simulink model "FuelCell"  (R2023a)
settings: Solver=VariableStepAuto  StartTime=0.0  StopTime=10  RelTol=1e-3
libraries: simulink x1, spspowerguiLib x1
settings Model: Creator=pc  LastModifiedBy=Faraz
settings DebuggingCC: ParameterPrecisionLossMsg=none

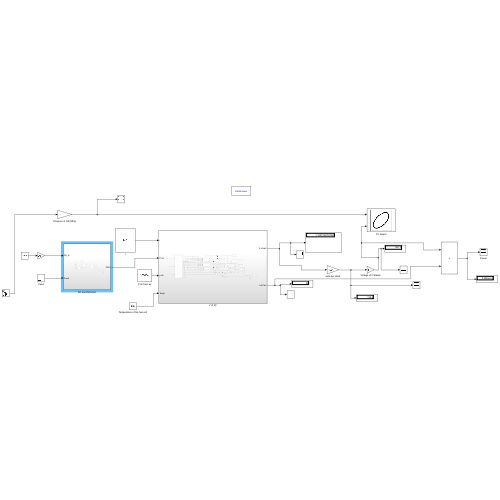
[thumbnail: Simulink's stored preview of the top-level diagram]
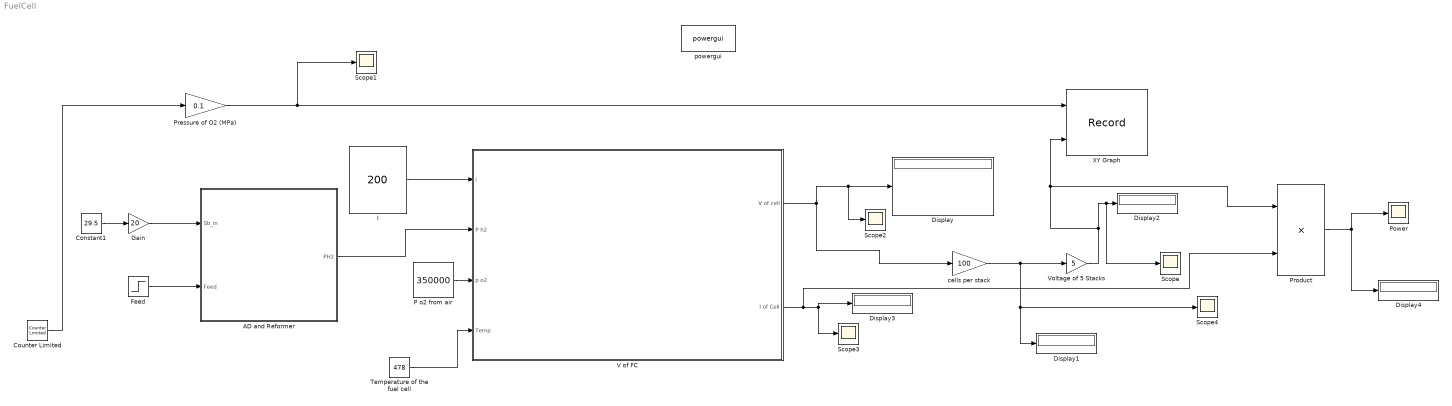
== system FuelCell ==
  AD and Reformer : Subsystem
  Constant1 : Constant  Value=29.5
  Counter Limited : simulink/Sources/Counter Limited  uplimit=50  tsamp=-1
  Display{,1..4} (5 alike) : Display
  Feed : Step  SampleTime=0
  Gain : Gain  Gain=20
  I : Constant  Value=200
  P o2 from air : Constant  Value=350000
  Power : Scope
  Pressure of O2 (MPa) : Gain  Gain=0.1
  Product : Product
  Scope{,1..4} (5 alike) : Scope
  Temperature of the fuel cell : Constant  Value=478
  V of FC : Subsystem
  Voltage of 5 Stacks : Gain  Gain=5
  XY Graph : Record  FileSettingsInternal="{\"entries\":[{\"content\":{\"excelSettings\":{\"content\":{},\"type\":\"Streamout.ExcelSettings\"}},\"type\":\"Streamout.FileSettingStorage\",\"uuid\":\"06980113-96f1-4b0c-a215-c6c45438d7ac\"}],\"packageUris\":[\"http://schema.mathworks.com/mf0/streamout_blocks/R2020a\"],\"version\":\"1.0\"}"  Layout=[1 1]  SignalsInternal="{\"entries\":[{\"content\":{\"signals\":[{\"content\":{\"blockPath\":[\"FuelCell/XY Graph\"],\"dimensions\":[1],\"domain\":\"FuelCell/XY Graph\",\"lineColor\":\"#a2142f\",\"plots\":[1],\"port\":1,\"sid\":[\"\"],\"signalID\":456,\"signalName\":\"Pressure of O2 (MPa)\"},\"type\":\"RecordBlkView.Signal\",\"uuid\":\"e1d00316-961b-4916-b371-07965f440cbd\"},{\"content\":{\"blockPath\":[\"FuelCell/XY Graph\"],\"dimensions\":[1],\"domain\":\"FuelCell/XY Graph\",\"lineColor\":\"#139fff\",\"plots\":[1],\"port\":2,\"sid\":[\"\"],\"signalID\":460,\"signalName\":\"Voltage of 5 Stacks\"},\"type\":\"RecordBlkView.Signal\",\"uuid\":\"8fd97479-0bd7-4bc4-89e8-e46443fea8dd\"}]},\"type\":\"RecordBlkView.InputSignals\",\"uuid\":\"3637481a-cae3-4c48-904e-6dbd072400be\"}],\"packageUris\":[\"http://schema.mathworks.com/mf0/streamout_blocks/R2020a\"],\"version\":\"1.0\"}"  VisualizationBindings="{\"xyplotplugin\":{\"info\":[{\"series\":[{\"bindingParametersList\":[{\"parameter\":\"X-Axis\",\"signalID\":456,\"signalName\":\"Pressure of O2 (MPa)\"},{\"parameter\":\"Y-Axis\",\"signalID\":460,\"signalName\":\"Voltage of 5 Stacks\"}],\"seriesID\":32857}],\"subplotID\":1}]}}"  CompatibilityTag=XY
  cells per stack : Gain  Gain=100
  powergui : spspowerguiLib/powergui  Priority=1  SimulationMode=Continuous  SampleTime=50e-6  frequency=60  Iterations=50  frequencyindice=0  Pbase=100e6  ErrMax=1e-4  UnitsV=kV  UnitsW=MW  buscounter=0  FunctionMessages=off  echomessages=off  EnableUseOfTLC=off  CurrentSourceSwitches=off  DisableSnubberDevices=off  DisableRonSwitches=off  DisableVfSwitches=off  DisplayEquations=off  AutomaticDiscreteSolvers=off  SolverType=Tustin/Backward Euler (TBE)  Interpol=off  ExternalGateDelay=off  methode=off  Ts=100  x0status=blocks  SPID=on  SwTol=0  HookPort=off  NonlinearTolerance=1e-4  nMaxIteration=100  ContinueOnMaxIteration=off  RestoreLinks=warning  ResistiveCurrentMeasurement=off  Frange=[0:2:500]  Ylog=off  Xlog=on  ShowGrid=off  save=off  variable=ZData  structure=0  ZoomFFT=off  StartTime=0.0  cycles=1  DisplayStyle=1  fundamental=60  FreqAxis=off  MaxFrequency=1000  frequencyindicesteady=1  RmsSteady=1  display=off
  wires:
  V of FC/1(V of cell) -> cells per stack/1, Scope2/1, Display/1
  I/1 -> V of FC/1("i ")
  cells per stack/1 -> Scope4/1, Display1/1, Voltage of 5 Stacks/1
  Voltage of 5 Stacks/1 -> Product/1, XY Graph/2, Scope/1, Display2/1
  Temperature of the fuel cell/1 -> V of FC/4(Temp)
  Counter Limited/1 -> Pressure of O2 (MPa)/1
  Pressure of O2 (MPa)/1 -> Scope1/1, XY Graph/1
  V of FC/2(I of Cell) -> Product/2, Display3/1, Scope3/1
  Gain/1 -> AD and Reformer/1(Sb_in)
  Constant1/1 -> Gain/1
  Feed/1 -> AD and Reformer/2(Feed)
  Product/1 -> Display4/1, Power/1
  AD and Reformer/1(PH2) -> V of FC/2(P h2)
  P o2 from air/1 -> V of FC/3(p o2)

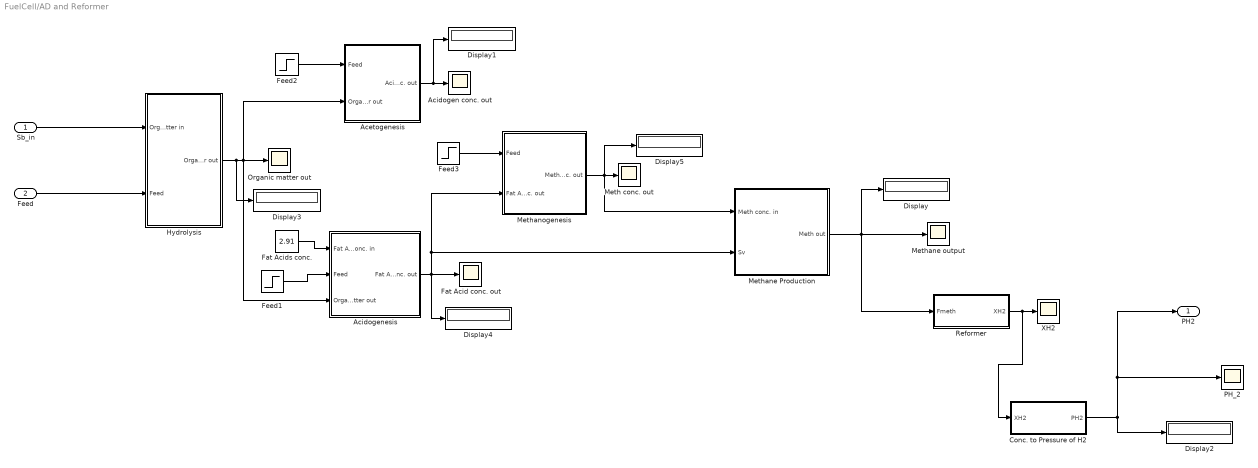
== system FuelCell/AD and Reformer ==
  Sb_in : Inport
  Feed : Inport  Port=2
  Acetogenesis : Subsystem
  Acidogen conc. out : Scope
  Acidogenesis : Subsystem
  Conc. to Pressure of H2 : Subsystem
  Display{,1..5} (6 alike) : Display
  Fat Acid conc. out : Scope
  Fat Acids conc. : Constant  Value=2.91
  Feed1 : Step  SampleTime=0
  Feed2 : Step  SampleTime=0
  Feed3 : Step  SampleTime=0
  "Hydrolysis " : Subsystem
  Meth conc. out : Scope
  Methane Production : Subsystem
  Methane output : Scope
  Methanogenesis : Subsystem
  Organic matter out : Scope
  PH_2 : Scope
  Reformer : Subsystem
  XH2 : Scope
  PH2 : Outport
  wires:
  Reformer/1(XH2) -> XH2/1, Conc. to Pressure of H2/1(XH2)
  Feed3/1 -> Methanogenesis/1(Feed)
  Feed1/1 -> Acidogenesis/2(Feed)
  Feed2/1 -> Acetogenesis/1(Feed)
  Acetogenesis/1(Acidogen conc. out) -> Display1/1, Acidogen conc. out/1
  Methanogenesis/1(Meth conc. out) -> Display5/1, Meth conc. out/1, Methane Production/1(Meth conc. in)
  Conc. to Pressure of H2/1(PH2) -> PH2/1, PH_2/1, Display2/1
  "Hydrolysis "/1(Organic matter out) -> Organic matter out/1, Acidogenesis/3(Organic matter out), Acetogenesis/2(Organic matter out), Display3/1
  Acidogenesis/1(Fat Acid conc. out) -> Display4/1, Methanogenesis/2(Fat Acid conc. out), Methane Production/2(Sv), Fat Acid conc. out/1
  Fat Acids conc./1 -> Acidogenesis/1(Fat Acid conc. in)
  Feed/1 -> "Hydrolysis "/2(Feed)
  Sb_in/1 -> "Hydrolysis "/1(Organic Matter in)
  Methane Production/1(Meth out) -> Methane output/1, Reformer/1(Fmeth), Display/1

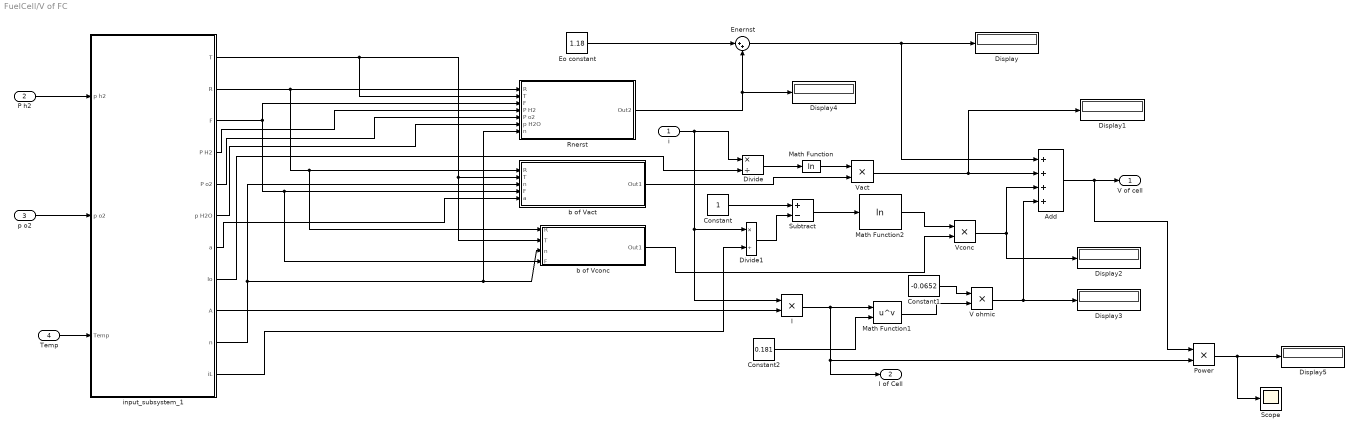
== system FuelCell/V of FC ==
  "i " : Inport
  P h2 : Inport  Port=2
  p o2 : Inport  Port=3
  Temp : Inport  Port=4
  Add : Sum  Inputs=++++
  Constant : Constant
  Constant1 : Constant  Value=-0.0652
  Constant2 : Constant  Value=0.181
  Display{,1..5} (6 alike) : Display
  Divide : Product  Inputs=*/
  Divide1 : Product  Inputs=*/
  Enernst : Sum  Inputs=|++
  "Eo constant " : Constant  Value=1.18
  I : Product
  Math Function : Math  Operator=log
  Math Function1 : Math  Operator=pow
  Math Function2 : Math  Operator=log
  Power : Product
  Rnerst : Subsystem
  Scope : Scope
  Subtract : Sum  Inputs=+-
  V ohmic : Product
  Vact : Product
  Vconc : Product
  b of Vact : Subsystem
  b of Vconc : Subsystem
  input_subsystem_1 : Subsystem
  V of cell : Outport
  I of Cell : Outport  Port=2
  wires:
  V ohmic/1 -> Display3/1, Add/4
  p o2/1 -> input_subsystem_1/2(p o2)
  input_subsystem_1/8(Io) -> Divide/2
  Temp/1 -> input_subsystem_1/3(Temp)
  P h2/1 -> input_subsystem_1/1(p h2)
  input_subsystem_1/11(iL) -> Divide1/2
  I/1 -> Math Function1/1, I of Cell/1, Power/2
  Enernst/1 -> Display/1, Add/1
  input_subsystem_1/9(A) -> I/2
  Vconc/1 -> Add/3, Display2/1
  input_subsystem_1/7(a) -> b of Vact/5(a)
  Math Function2/1 -> Vconc/1
  Constant2/1 -> Math Function1/2
  "i "/1 -> Divide/1, Divide1/1, I/1
  "Eo constant "/1 -> Enernst/1
  input_subsystem_1/5(P o2) -> Rnerst/5(P o2)
  b of Vconc/1(Out1) -> Vconc/2
  Subtract/1 -> Math Function2/1
  input_subsystem_1/6(p H2O) -> Rnerst/6(p H2O)
  input_subsystem_1/4(P H2) -> Rnerst/4(P H2)
  Constant/1 -> Subtract/1
  b of Vact/1(Out1) -> Vact/2
  Rnerst/1(Out2) -> Enernst/2, Display4/1
  Vact/1 -> Add/2, Display1/1
  Math Function/1 -> Vact/1
  Divide/1 -> Math Function/1
  input_subsystem_1/1(T) -> b of Vconc/2(T), b of Vact/2(T), Rnerst/2(T)
  Math Function1/1 -> V ohmic/2
  input_subsystem_1/2(R) -> Rnerst/1(R), b of Vconc/1(R), b of Vact/1(R)
  Add/1 -> V of cell/1, Power/1
  Divide1/1 -> Subtract/2
  Constant1/1 -> V ohmic/1
  Power/1 -> Scope/1, Display5/1
  input_subsystem_1/3(F) -> b of Vconc/4(F), b of Vact/4(F), Rnerst/3(F)
  input_subsystem_1/10(n) -> b of Vact/3(n), b of Vconc/3(n), Rnerst/7(n)

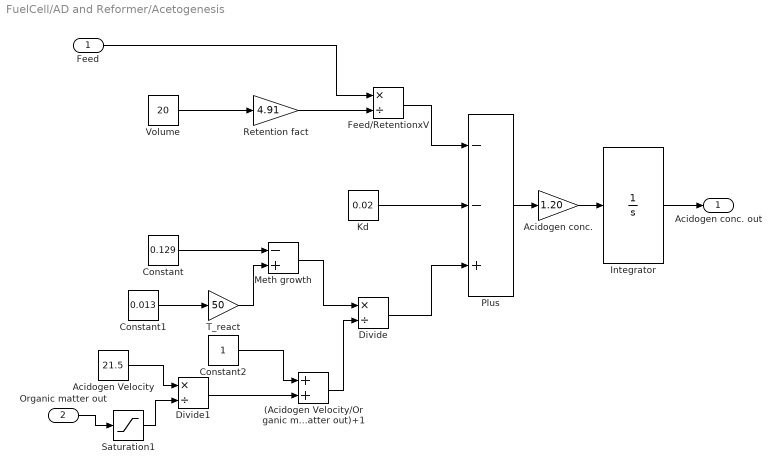
== system FuelCell/AD and Reformer/Acetogenesis ==
  Feed : Inport
  Organic matter out : Inport  Port=2
  (Acidogen Velocity/Organic matter out)+1 : Sum
  Acidogen Velocity : Constant  Value=21.5
  Acidogen conc. : Gain  Gain=1.20
  Constant : Constant  Value=0.129
  Constant1 : Constant  Value=0.013
  Constant2 : Constant
  Divide : Product  Inputs=*/
  Divide1 : Product  Inputs=*/
  Feed/RetentionxV : Product  Inputs=*/
  Integrator : Integrator
  Kd : Constant  Value=0.02
  Meth growth : Sum  Inputs=-+
  Plus : Sum  Inputs=--+
  Retention fact : Gain  Gain=4.91
  Saturation1 : Saturate  UpperLimit=300  LowerLimit=0.3
  T_react : Gain  Gain=50
  Volume : Constant  Value=20
  Acidogen conc. out : Outport
  wires:
  Volume/1 -> Retention fact/1
  Retention fact/1 -> Feed/RetentionxV/2
  Feed/1 -> Feed/RetentionxV/1
  Feed/RetentionxV/1 -> Plus/1
  Kd/1 -> Plus/2
  Acidogen conc./1 -> Integrator/1
  Plus/1 -> Acidogen conc./1
  Constant1/1 -> T_react/1
  T_react/1 -> Meth growth/2
  Constant/1 -> Meth growth/1
  Meth growth/1 -> Divide/1
  (Acidogen Velocity/Organic matter out)+1/1 -> Divide/2
  Constant2/1 -> (Acidogen Velocity/Organic matter out)+1/1
  Acidogen Velocity/1 -> Divide1/1
  Divide/1 -> Plus/3
  Integrator/1 -> Acidogen conc. out/1
  Organic matter out/1 -> Saturation1/1
  Divide1/1 -> (Acidogen Velocity/Organic matter out)+1/2
  Saturation1/1 -> Divide1/2

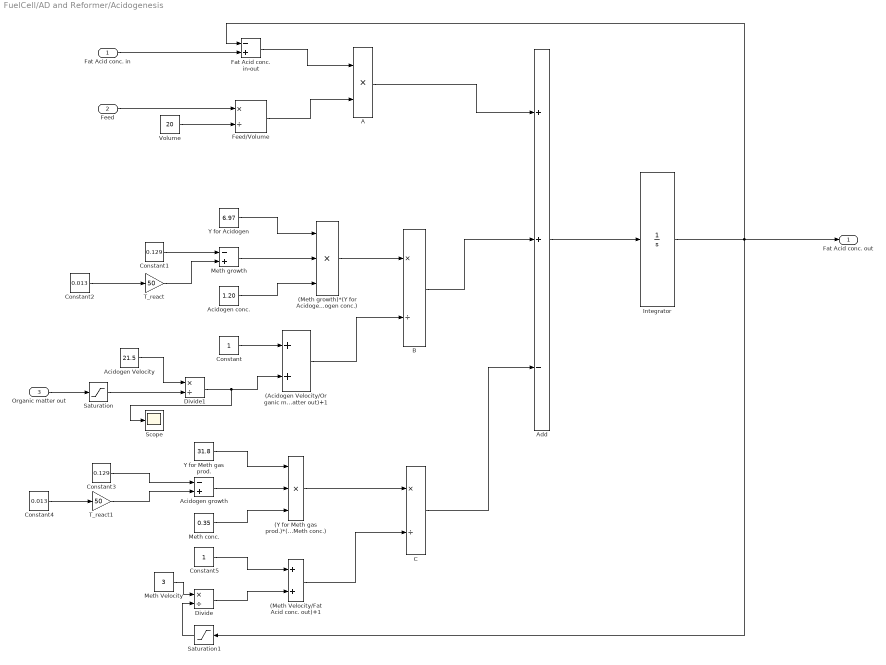
== system FuelCell/AD and Reformer/Acidogenesis ==
  Fat Acid conc. in : Inport
  Feed : Inport  Port=2
  Organic matter out : Inport  Port=3
  (Acidogen Velocity/Organic matter out)+1 : Sum
  (Meth Velocity/Fat Acid conc. out)+1 : Sum
  (Meth growth)*(Y for Acidogen)*(Acidogen conc.) : Product  Inputs=3
  (Y for Meth gas prod.)*(Acid growth)*(Meth conc.) : Product  Inputs=3
  A : Product
  Acidogen Velocity : Constant  Value=21.5
  Acidogen conc. : Constant  Value=1.20
  Acidogen growth : Sum  Inputs=-+
  Add : Sum  Inputs=++-
  B : Product  Inputs=*/
  C : Product  Inputs=*/
  Constant : Constant
  Constant1 : Constant  Value=0.129
  Constant2 : Constant  Value=0.013
  Constant3 : Constant  Value=0.129
  Constant4 : Constant  Value=0.013
  Constant5 : Constant
  Divide : Product  Inputs=*/
  Divide1 : Product  Inputs=*/
  Fat Acid conc. in-out : Sum  Inputs=-+
  Feed/Volume : Product  Inputs=*/
  Integrator : Integrator
  Meth Velocity : Constant  Value=3
  Meth conc. : Constant  Value=0.35
  Meth growth : Sum  Inputs=-+
  Saturation : Saturate  UpperLimit=100  LowerLimit=0.002
  Saturation1 : Saturate  UpperLimit=300  LowerLimit=0.3
  Scope : Scope
  T_react : Gain  Gain=50
  T_react1 : Gain  Gain=50
  Volume : Constant  Value=20
  Y for Acidogen : Constant  Value=6.97
  Y for Meth gas prod. : Constant  Value=31.8
  Fat Acid conc. out : Outport
  wires:
  Integrator/1 -> Saturation1/1, Fat Acid conc. in-out/1, Fat Acid conc. out/1
  Fat Acid conc. in/1 -> Fat Acid conc. in-out/2
  Feed/1 -> Feed/Volume/1
  Fat Acid conc. in-out/1 -> A/1
  Feed/Volume/1 -> A/2
  Volume/1 -> Feed/Volume/2
  A/1 -> Add/1
  (Meth growth)*(Y for Acidogen)*(Acidogen conc.)/1 -> B/1
  B/1 -> Add/2
  (Acidogen Velocity/Organic matter out)+1/1 -> B/2
  Meth growth/1 -> (Meth growth)*(Y for Acidogen)*(Acidogen conc.)/2
  Y for Acidogen/1 -> (Meth growth)*(Y for Acidogen)*(Acidogen conc.)/1
  Constant1/1 -> Meth growth/1
  Acidogen conc./1 -> (Meth growth)*(Y for Acidogen)*(Acidogen conc.)/3
  Divide1/1 -> Scope/1, (Acidogen Velocity/Organic matter out)+1/2
  T_react/1 -> Meth growth/2
  Constant2/1 -> T_react/1
  Constant/1 -> (Acidogen Velocity/Organic matter out)+1/1
  Acidogen Velocity/1 -> Divide1/1
  Add/1 -> Integrator/1
  C/1 -> Add/3
  (Y for Meth gas prod.)*(Acid growth)*(Meth conc.)/1 -> C/1
  Acidogen growth/1 -> (Y for Meth gas prod.)*(Acid growth)*(Meth conc.)/2
  (Meth Velocity/Fat Acid conc. out)+1/1 -> C/2
  Divide/1 -> (Meth Velocity/Fat Acid conc. out)+1/2
  Y for Meth gas prod./1 -> (Y for Meth gas prod.)*(Acid growth)*(Meth conc.)/1
  Constant3/1 -> Acidogen growth/1
  T_react1/1 -> Acidogen growth/2
  Constant4/1 -> T_react1/1
  Meth conc./1 -> (Y for Meth gas prod.)*(Acid growth)*(Meth conc.)/3
  Constant5/1 -> (Meth Velocity/Fat Acid conc. out)+1/1
  Meth Velocity/1 -> Divide/1
  Organic matter out/1 -> Saturation/1
  Saturation/1 -> Divide1/2
  Saturation1/1 -> Divide/2

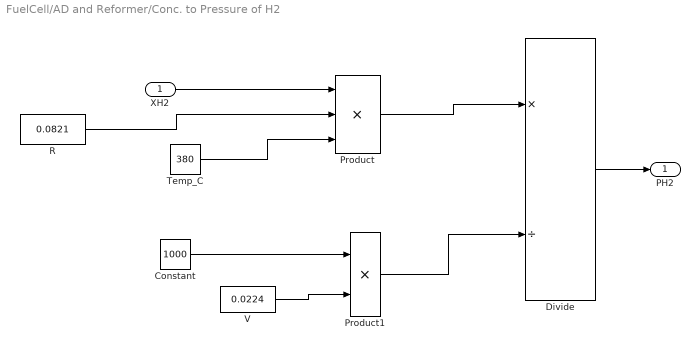
== system FuelCell/AD and Reformer/Conc. to Pressure of H2 ==
  XH2 : Inport
  Constant : Constant  Value=1000
  Divide : Product  Inputs=*/
  Product : Product  Inputs=3
  Product1 : Product
  R : Constant  Value=0.0821
  Temp_C : Constant  Value=380
  V : Constant  Value=0.0224
  PH2 : Outport
  wires:
  XH2/1 -> Product/1
  R/1 -> Product/2
  Temp_C/1 -> Product/3
  Constant/1 -> Product1/1
  V/1 -> Product1/2
  Product1/1 -> Divide/2
  Product/1 -> Divide/1
  Divide/1 -> PH2/1

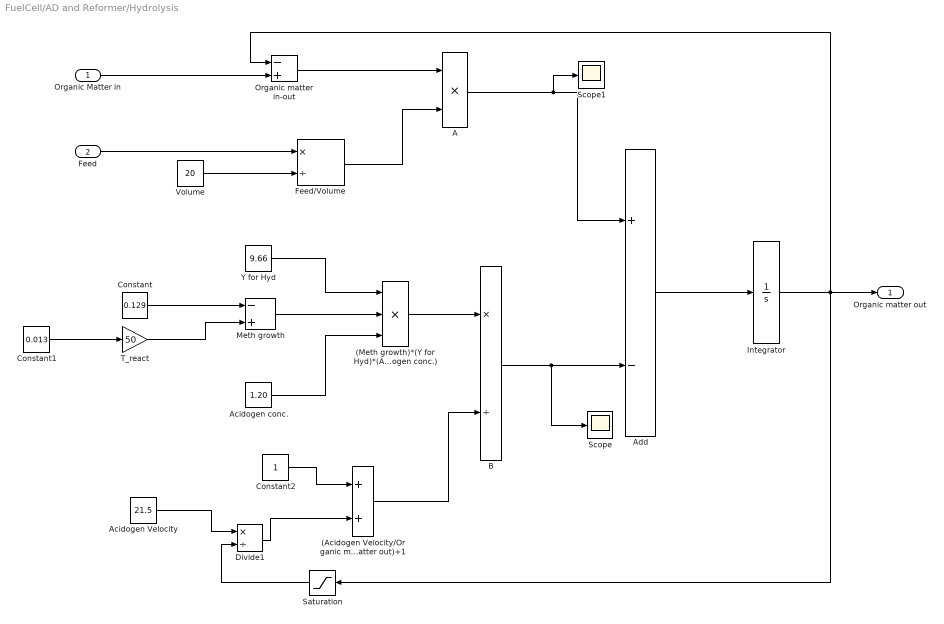
== system FuelCell/AD and Reformer/Hydrolysis  ==
  Organic Matter in : Inport
  Feed : Inport  Port=2
  (Acidogen Velocity/Organic matter out)+1 : Sum
  (Meth growth)*(Y for Hyd)*(Acidogen conc.) : Product  Inputs=3
  A : Product
  Acidogen Velocity : Constant  Value=21.5
  Acidogen conc. : Constant  Value=1.20
  Add : Sum  Inputs=+-
  B : Product  Inputs=*/
  Constant : Constant  Value=0.129
  Constant1 : Constant  Value=0.013
  Constant2 : Constant
  Divide1 : Product  Inputs=*/
  Feed/Volume : Product  Inputs=*/
  Integrator : Integrator
  Meth growth : Sum  Inputs=-+
  Organic matter in-out : Sum  Inputs=-+
  Saturation : Saturate  UpperLimit=300  LowerLimit=0.3
  Scope : Scope
  Scope1 : Scope
  T_react : Gain  Gain=50
  Volume : Constant  Value=20
  Y for Hyd : Constant  Value=9.66
  Organic matter out : Outport
  wires:
  Feed/1 -> Feed/Volume/1
  Organic Matter in/1 -> Organic matter in-out/2
  Volume/1 -> Feed/Volume/2
  Constant/1 -> Meth growth/1
  Constant1/1 -> T_react/1
  T_react/1 -> Meth growth/2
  Organic matter in-out/1 -> A/1
  Feed/Volume/1 -> A/2
  A/1 -> Scope1/1, Add/1
  Y for Hyd/1 -> (Meth growth)*(Y for Hyd)*(Acidogen conc.)/1
  Meth growth/1 -> (Meth growth)*(Y for Hyd)*(Acidogen conc.)/2
  Acidogen conc./1 -> (Meth growth)*(Y for Hyd)*(Acidogen conc.)/3
  (Meth growth)*(Y for Hyd)*(Acidogen conc.)/1 -> B/1
  Acidogen Velocity/1 -> Divide1/1
  Constant2/1 -> (Acidogen Velocity/Organic matter out)+1/1
  (Acidogen Velocity/Organic matter out)+1/1 -> B/2
  B/1 -> Scope/1, Add/2
  Integrator/1 -> Saturation/1, Organic matter in-out/1, Organic matter out/1
  Add/1 -> Integrator/1
  Divide1/1 -> (Acidogen Velocity/Organic matter out)+1/2
  Saturation/1 -> Divide1/2

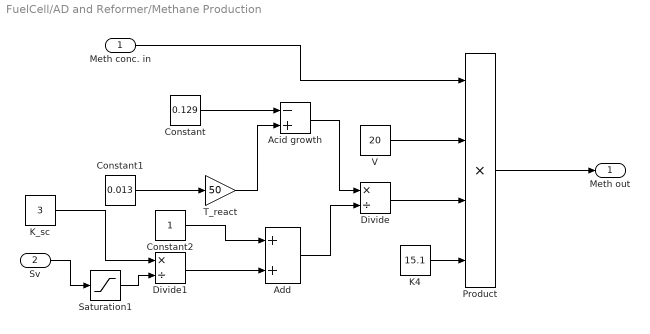
== system FuelCell/AD and Reformer/Methane Production ==
  Meth conc. in : Inport
  Sv : Inport  Port=2
  Acid growth : Sum  Inputs=-+
  Add : Sum
  Constant : Constant  Value=0.129
  Constant1 : Constant  Value=0.013
  Constant2 : Constant
  Divide : Product  Inputs=*/
  Divide1 : Product  Inputs=*/
  K4 : Constant  Value=15.1
  K_sc : Constant  Value=3
  Product : Product  Inputs=4
  Saturation1 : Saturate  UpperLimit=100  LowerLimit=0.3
  T_react : Gain  Gain=50
  V : Constant  Value=20
  Meth out : Outport
  wires:
  T_react/1 -> Acid growth/2
  Constant/1 -> Acid growth/1
  V/1 -> Product/2
  Constant1/1 -> T_react/1
  Meth conc. in/1 -> Product/1
  K4/1 -> Product/4
  Product/1 -> Meth out/1
  Divide/1 -> Product/3
  Acid growth/1 -> Divide/1
  K_sc/1 -> Divide1/1
  Sv/1 -> Saturation1/1
  Divide1/1 -> Add/2
  Constant2/1 -> Add/1
  Add/1 -> Divide/2
  Saturation1/1 -> Divide1/2

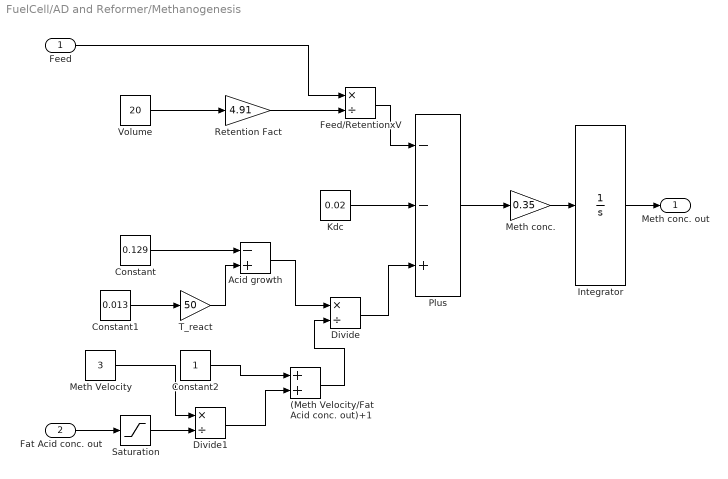
== system FuelCell/AD and Reformer/Methanogenesis ==
  Feed : Inport
  Fat Acid conc. out : Inport  Port=2
  (Meth Velocity/Fat Acid conc. out)+1 : Sum
  Acid growth : Sum  Inputs=-+
  Constant : Constant  Value=0.129
  Constant1 : Constant  Value=0.013
  Constant2 : Constant
  Divide : Product  Inputs=*/
  Divide1 : Product  Inputs=*/
  "Feed/RetentionxV " : Product  Inputs=*/
  Integrator : Integrator
  Kdc : Constant  Value=0.02
  Meth Velocity : Constant  Value=3
  Meth conc. : Gain  Gain=0.35
  Plus : Sum  Inputs=--+
  Retention Fact : Gain  Gain=4.91
  Saturation : Saturate  UpperLimit=300  LowerLimit=0.3
  T_react : Gain  Gain=50
  Volume : Constant  Value=20
  Meth conc. out : Outport
  wires:
  Divide/1 -> Plus/3
  T_react/1 -> Acid growth/2
  Constant/1 -> Acid growth/1
  Divide1/1 -> (Meth Velocity/Fat Acid conc. out)+1/2
  Fat Acid conc. out/1 -> Saturation/1
  Kdc/1 -> Plus/2
  Constant2/1 -> (Meth Velocity/Fat Acid conc. out)+1/1
  Feed/1 -> "Feed/RetentionxV "/1
  Volume/1 -> Retention Fact/1
  (Meth Velocity/Fat Acid conc. out)+1/1 -> Divide/2
  Meth Velocity/1 -> Divide1/1
  Constant1/1 -> T_react/1
  Integrator/1 -> Meth conc. out/1
  Acid growth/1 -> Divide/1
  Meth conc./1 -> Integrator/1
  Retention Fact/1 -> "Feed/RetentionxV "/2
  "Feed/RetentionxV "/1 -> Plus/1
  Plus/1 -> Meth conc./1
  Saturation/1 -> Divide1/2

== system FuelCell/AD and Reformer/Reformer ==
  Fmeth : Inport
  Concentration of Hot H2O (exp) : Constant  Value=980
  Gain : Gain  Gain=3
  Product : Product  Inputs=3
  Rate constant for SMR : Constant  Value=2.1
  XH2 : Outport
  wires:
  Fmeth/1 -> Product/1
  Rate constant for SMR/1 -> Gain/1
  Gain/1 -> Product/2
  Product/1 -> XH2/1
  Concentration of Hot H2O (exp)/1 -> Product/3

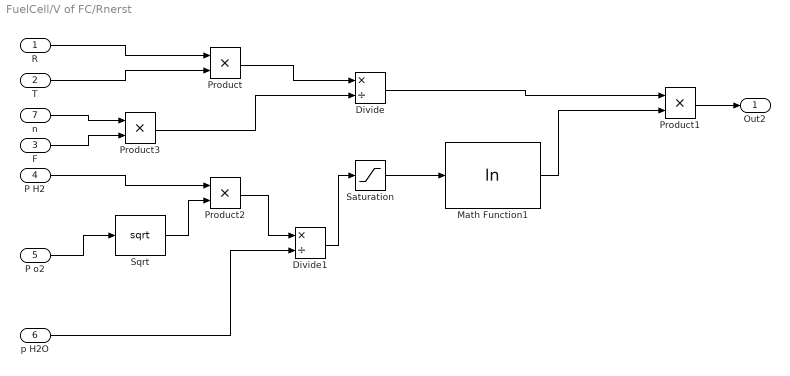
== system FuelCell/V of FC/Rnerst ==
  R : Inport
  T : Inport  Port=2
  F : Inport  Port=3
  P H2 : Inport  Port=4
  P o2 : Inport  Port=5
  p H2O : Inport  Port=6
  n : Inport  Port=7
  Divide : Product  Inputs=*/
  Divide1 : Product  Inputs=*/
  Math Function1 : Math  Operator=log
  Product{,1..3} (4 alike) : Product
  Saturation : Saturate  UpperLimit=100000000  LowerLimit=0.005
  Sqrt : Sqrt
  Out2 : Outport
  wires:
  p H2O/1 -> Divide1/2
  Product2/1 -> Divide1/1
  Product3/1 -> Divide/2
  F/1 -> Product3/2
  n/1 -> Product3/1
  T/1 -> Product/2
  R/1 -> Product/1
  Product/1 -> Divide/1
  Divide/1 -> Product1/1
  P H2/1 -> Product2/1
  P o2/1 -> Sqrt/1
  Sqrt/1 -> Product2/2
  Math Function1/1 -> Product1/2
  Product1/1 -> Out2/1
  Divide1/1 -> Saturation/1
  Saturation/1 -> Math Function1/1

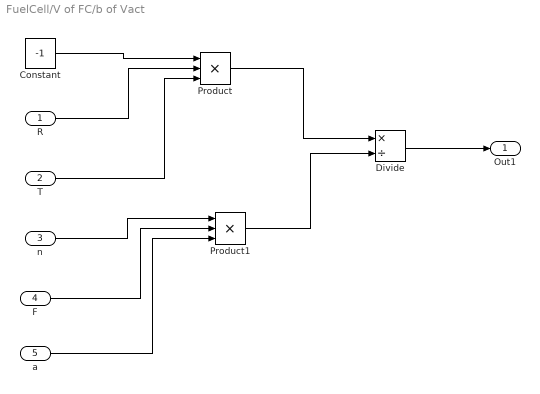
== system FuelCell/V of FC/b of Vact ==
  R : Inport
  T : Inport  Port=2
  n : Inport  Port=3
  F : Inport  Port=4
  a : Inport  Port=5
  Constant : Constant  Value=-1
  Divide : Product  Inputs=*/
  Product : Product  Inputs=3
  Product1 : Product  Inputs=3
  Out1 : Outport
  wires:
  Constant/1 -> Product/1
  R/1 -> Product/2
  T/1 -> Product/3
  n/1 -> Product1/1
  F/1 -> Product1/2
  a/1 -> Product1/3
  Product/1 -> Divide/1
  Product1/1 -> Divide/2
  Divide/1 -> Out1/1

== system FuelCell/V of FC/b of Vconc ==
  R : Inport
  T : Inport  Port=2
  n : Inport  Port=3
  F : Inport  Port=4
  Divide : Product  Inputs=*/
  Product : Product
  Product1 : Product
  Out1 : Outport
  wires:
  R/1 -> Product/1
  T/1 -> Product/2
  n/1 -> Product1/1
  F/1 -> Product1/2
  Product/1 -> Divide/1
  Product1/1 -> Divide/2
  Divide/1 -> Out1/1

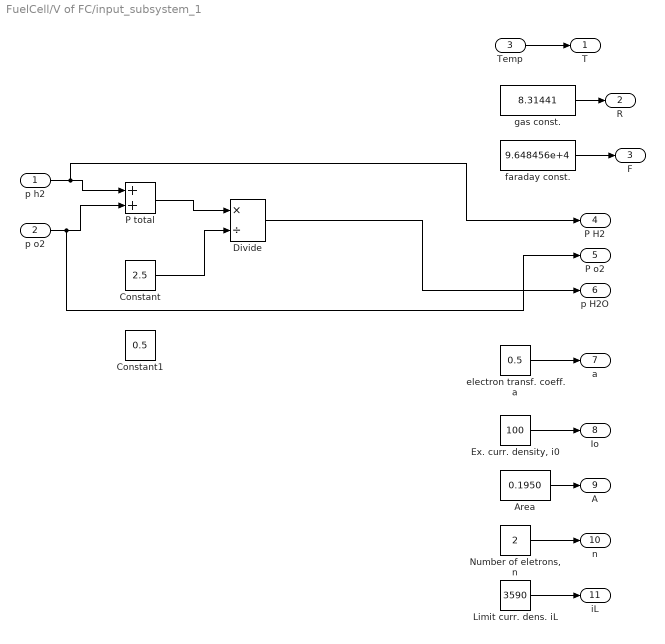
== system FuelCell/V of FC/input_subsystem_1 ==
  p h2 : Inport
  p o2 : Inport  Port=2
  Temp : Inport  Port=3
  Area : Constant  Value=0.1950
  Constant : Constant  Value=2.5
  Constant1 : Constant  Value=0.5
  Divide : Product  Inputs=*/
  "Ex. curr. density, i0" : Constant  Value=100
  Limit curr. dens. iL : Constant  Value=3590
  "Number of eletrons, n" : Constant  Value=2
  P total : Sum
  electron transf. coeff. a : Constant  Value=0.5
  faraday const. : Constant  Value=9.648456e+4
  gas const. : Constant  Value=8.31441
  T : Outport
  R : Outport  Port=2
  F : Outport  Port=3
  P H2 : Outport  Port=4
  P o2 : Outport  Port=5
  p H2O : Outport  Port=6
  a : Outport  Port=7
  Io : Outport  Port=8
  A : Outport  Port=9
  n : Outport  Port=10
  iL : Outport  Port=11
  wires:
  p o2/1 -> P o2/1, P total/2
  Divide/1 -> p H2O/1
  Constant/1 -> Divide/2
  P total/1 -> Divide/1
  p h2/1 -> P H2/1, P total/1
  gas const./1 -> R/1
  Temp/1 -> T/1
  faraday const./1 -> F/1
  "Number of eletrons, n"/1 -> n/1
  Area/1 -> A/1
  electron transf. coeff. a/1 -> a/1
  "Ex. curr. density, i0"/1 -> Io/1
  Limit curr. dens. iL/1 -> iL/1
